simulink model "E0_Calculate"  (R2020a)
settings: Solver=VariableStepAuto  StartTime=0.0  StopTime=10.0  RelTol=1e-3
values from neighbouring files (symbols this model uses):
  Z1 = complex(R1, X1)    [para.m]    (also in parameter.m)
settings Model: Creator=EPESL  LastModifiedBy=EPESL

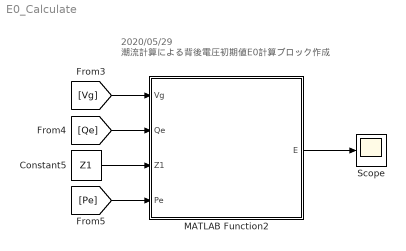
== system E0_Calculate ==
  note: 2020/05/29
      | 潮流計算による背後電圧初期値E0計算ブロック作成
  Constant5 : Constant  Value=Z1
  MATLAB Function2 : MATLAB Function  TreatAsAtomicUnit=on
  Scope : Scope
  wires:
  MATLAB Function2/1(E) -> Scope/1
  [Qe] -> MATLAB Function2/2(Qe)
  Constant5/1 -> MATLAB Function2/3(Z1)
  [Pe] -> MATLAB Function2/4(Pe)
  [Vg] -> MATLAB Function2/1(Vg)

== matlab function E0_Calculate/MATLAB Function2 ==
  data: Vg input; E output; Qe input; Z1 input; Pe input
function E = fcn(Vg,Qe,Z1,Pe)

E = (Vg+Qe*Z1/Vg)+1i*(Pe*Z1/Vg);
